simulink model "elevator_ISE"  (R2017b)
settings: Solver=VariableStepAuto  StartTime=0.0  StopTime=10  RelTol=1e-3
values from neighbouring files (symbols this model uses):
  D = 9    [mfile_IAE.m]
  G_ol = Torque*G    [mfile_IAE.m]
  k = [1 1 1]    [mfile_IAE.m]
  w = pi/10    (= 0.314159265359)    [mfile_IAE.m]
settings Model: Creator=sara  LastModifiedBy=sara

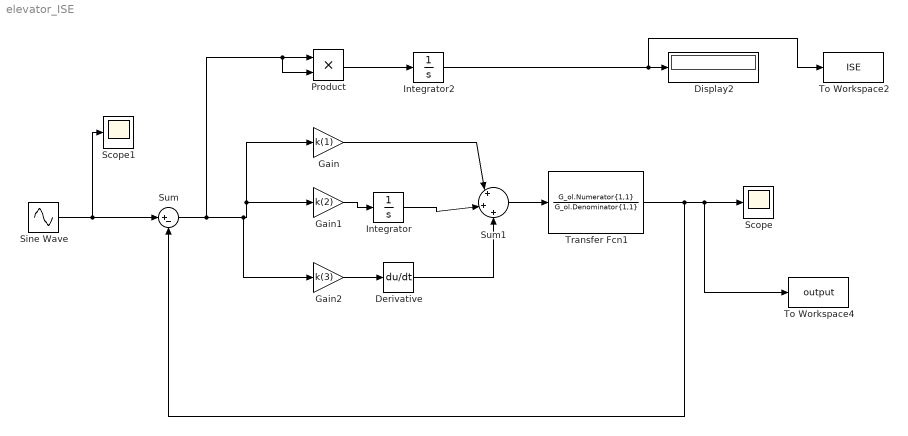
== system elevator_ISE ==
  Derivative : Derivative
  Display2 : Display
  Gain : Gain  Gain=k(1)
  Gain1 : Gain  Gain=k(2)
  Gain2 : Gain  Gain=k(3)
  Integrator : Integrator
  Integrator2 : Integrator
  Product : Product
  Scope : Scope
  Scope1 : Scope
  Sine Wave : Sin  Amplitude=-D/2  Bias=D/2  Frequency=w  Phase=pi/2  SampleTime=0
  Sum : Sum  Inputs=|+-
  Sum1 : Sum  Inputs=|+|+|+
  To Workspace2 : ToWorkspace  VariableName=ISE  SampleTime=-1
      settings: Save2DSignal=2-D array (concatenate along first dimension)
  To Workspace4 : ToWorkspace  VariableName=output  SampleTime=-1
      settings: Save2DSignal=2-D array (concatenate along first dimension)
  Transfer Fcn1 : TransferFcn  Numerator=G_ol.Numerator{1,1}  Denominator=G_ol.Denominator{1,1}
  wires:
  Sine Wave/1 -> Scope1/1, Sum/1
  Gain/1 -> Sum1/1
  Integrator/1 -> Sum1/2
  Derivative/1 -> Sum1/3
  Gain2/1 -> Derivative/1
  Gain1/1 -> Integrator/1
  Sum/1 -> Product/2, Product/1, Gain2/1, Gain1/1, Gain/1
  Sum1/1 -> Transfer Fcn1/1
  Transfer Fcn1/1 -> To Workspace4/1, Scope/1, Sum/2
  Product/1 -> Integrator2/1
  Integrator2/1 -> To Workspace2/1, Display2/1
